simulink model "subsampling1"  (R2021a)
settings: Solver=VariableStepAuto  StartTime=0.0  StopTime=1  MaxStep=1/1e6  RelTol=1e-3
values from neighbouring files (symbols this model uses):
  fnoise = 1e6    (= 1000000)    [subsampling_1.m]    (also in subsampling_2.m; subsampling_3.m = 3000000; unterabtastung_1.m; unterabtastung_2.m)
  fs = 18e3    (= 18000)    [subsampling_1.m]    (also in subsampling_2.m; subsampling_3.m = 450000; unterabtastung_1.m; unterabtastung_2.m)
  fsin = 39e3    (= 39000)    [subsampling_1.m]    (also in subsampling_2.m; subsampling_3.m = 980000; unterabtastung_1.m; unterabtastung_2.m)
undefined symbols (not defined in the file or in its folder): a, b
libraries: simulink x1, dspsigops x1
settings Model: Creator=josef  LastModifiedBy=josef
settings SolverCC: AlgebraicLoopSolver=TrustRegion
settings DataIOCC: ReturnWorkspaceOutputs=off
settings DebuggingCC: SFMachineParentedDataDiag=warning

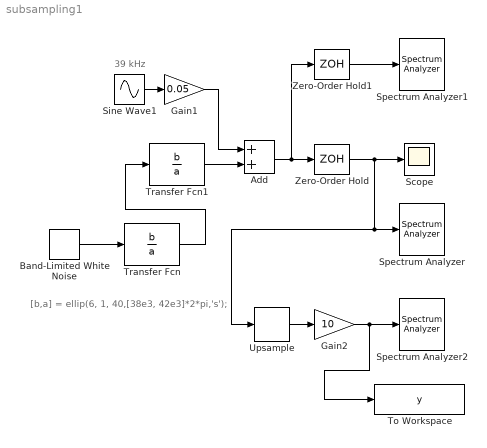
== system subsampling1 ==
  note: [b,a] = ellip(6, 1, 40,[38e3, 42e3]*2*pi,'s');
  note: 39 kHz
  Add : Sum
  Band-Limited White Noise : simulink/Sources/Band-Limited White Noise  Cov=1/fnoise  Ts=1/fnoise  seed=[23341]
  Gain1 : Gain  Gain=0.05
  Gain2 : Gain  Gain=10
  Scope : Scope
  Sine Wave1 : Sin  Frequency=2*pi*fsin  SampleTime=0
  Spectrum Analyzer : SpectrumAnalyzer
  Spectrum Analyzer1 : SpectrumAnalyzer
  Spectrum Analyzer2 : SpectrumAnalyzer
  To Workspace : ToWorkspace  VariableName=y  SaveFormat=Timeseries  SampleTime=-1
  Transfer Fcn : TransferFcn  Numerator=b  Denominator=a
  Transfer Fcn1 : TransferFcn  Numerator=b  Denominator=a
  Upsample : dspsigops/Upsample  N=10  phase=0  RateOptions=Allow multirate processing  ic=0  mode=Unused parameter value
  Zero-Order Hold : ZeroOrderHold  SampleTime=1/fs
  Zero-Order Hold1 : ZeroOrderHold  SampleTime=1/(10*fs)
  wires:
  Sine Wave1/1 -> Gain1/1
  Add/1 -> Zero-Order Hold1/1, Zero-Order Hold/1
  Gain1/1 -> Add/1
  Zero-Order Hold/1 -> Upsample/1, Spectrum Analyzer/1, Scope/1
  Zero-Order Hold1/1 -> Spectrum Analyzer1/1
  Band-Limited White Noise/1 -> Transfer Fcn/1
  Transfer Fcn/1 -> Transfer Fcn1/1
  Transfer Fcn1/1 -> Add/2
  Upsample/1 -> Gain2/1
  Gain2/1 -> To Workspace/1, Spectrum Analyzer2/1
